simulink model "Main_ekart"  (R2021b)
settings: Solver=FixedStepAuto  StartTime=0.0  StopTime=inf  FixedStep=1/500  RelTol=1e-3  EnableMultiTasking=on
values from neighbouring files (symbols this model uses):
  a = [1 -2.62355180661 2.31468258109 -0.685535977285]    [IMU_filt_100Hz.mat]    (also in IMU_filt_500Hz.mat = [1 -2.92460623545 2.85202781859 -0.92736996835])
  angles = [0 4.9 5 10 15 20 25 30 35 40]    [CreateAllControllers.m]
  b = [0.000699349649901 0.0020980489497 0.0020980489497 0.000699349649901]    [IMU_filt_100Hz.mat]    (also in IMU_filt_500Hz.mat = [6.45184912909e-06 1.93555473873e-05 1.93555473873e-05 6.451)
  D = (DMFx+DMFy)/2    (= 1.2194)    [kart_parameters2.m]
  gear_ratio = 3.2    [kart_parameters2.m]
  L = sys*C    [build_controller_PI.m]    (also in kart_parameters2.m = 1.042)
  newcurrent = [-186.423 -186.283922965 -186.14484593 -186.005768895 -185.866691861 -185.727614826 -185.588537791 -185.449460756 -185.310383721 -185.171306686 -185.032229652 -184.893152617 ... (1000 elements, 1x1000)]    [Torque_map.mat]
  newtorque = [-28.1755 -28.1190925926 -28.0626851852 -28.0062777778 -27.9498703704 -27.893462963 -27.8370555556 -27.7806481481 -27.7242407407 -27.6678333333 -27.6114259259 -27.5550185185 ... (1000 elements, 1x1000)]    [Torque_map.mat]
  percent = [0 0.1001001001 0.2002002002 0.3003003003 0.4004004004 0.500500500501 0.600600600601 0.700700700701 0.800800800801 0.900900900901 1.001001001 1.1011011011 ... (1000 elements, 1x1000)]    [Torque_accel.mat]
  speeds = [0 19.9 20 30 40]    [CreateAllControllers.m]
  table_i = [zeros(1,10) ... (first row only)    [CreateAllControllers.m]
  table_p = [zeros(1, 10) ... (first row only)    [CreateAllControllers.m]
  torque = [0.1025 0.130601101101 0.158702202202 0.186803303303 0.214904404404 0.243005505506 0.271106606607 0.299207707708 0.327308808809 0.35540990991 0.383511011011 0.411612112112 ... (1000 elements, 1x1000)]    [Torque_accel.mat]
libraries: simulink x50, mcp2515lib x46, etargetslib x4, svdutilitieslib x3, cstblocks x2, slpidlib x1
(part 4 of 4)

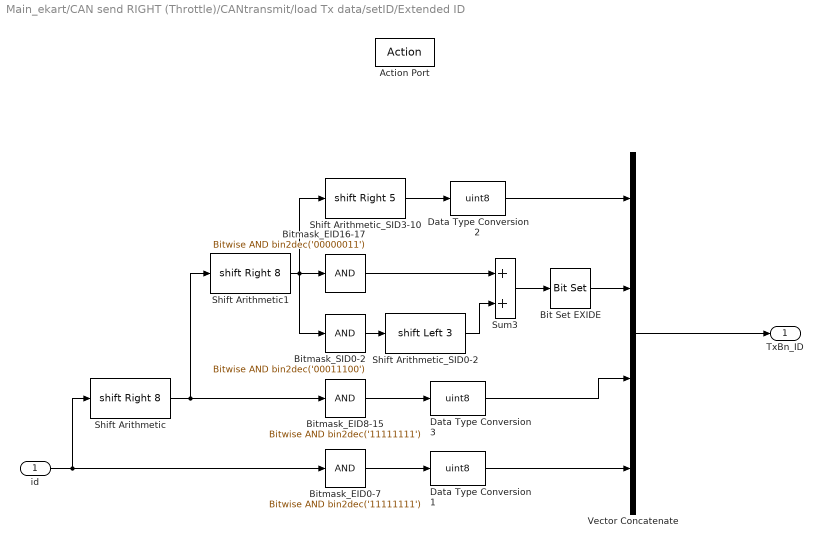
== system Main_ekart/CAN send RIGHT (Throttle)/CANtransmit/load Tx data/setID/Extended ID ==
  id : Inport
  Action Port : ActionPort  ActionPortLabel=if(u1 > 0)
  Bit Set EXIDE : simulink/Logic and Bit Operations/Bit Set  iBit=3
      settings: SourceProductBaseCode=SL
  Bitmask_EID0-7 : simulink/Logic and Bit Operations/Bitwise Operator  logicop=AND  UseBitMask=on  BitMask=bin2dec('11111111')  BitMaskRealWorld=Stored Integer
  Bitmask_EID16-17 : simulink/Logic and Bit Operations/Bitwise Operator  logicop=AND  UseBitMask=on  BitMask=bin2dec('00000011')  BitMaskRealWorld=Stored Integer
  Bitmask_EID8-15 : simulink/Logic and Bit Operations/Bitwise Operator  logicop=AND  UseBitMask=on  BitMask=bin2dec('11111111')  BitMaskRealWorld=Stored Integer
  Bitmask_SID0-2 : simulink/Logic and Bit Operations/Bitwise Operator  logicop=AND  UseBitMask=on  BitMask=bin2dec('00011100')  BitMaskRealWorld=Stored Integer
  Data Type Conversion1 : DataTypeConversion  OutDataTypeStr=uint8  RndMeth=Simplest
  Data Type Conversion2 : DataTypeConversion  OutDataTypeStr=uint8  RndMeth=Simplest
  Data Type Conversion3 : DataTypeConversion  OutDataTypeStr=uint8  RndMeth=Simplest
  Shift Arithmetic : ArithShift  BitShiftNumber=8  BitShiftDirection=Right
  Shift Arithmetic1 : ArithShift  BitShiftNumber=8  BitShiftDirection=Right
  Shift Arithmetic_SID0-2 : ArithShift  BitShiftNumber=3  BitShiftDirection=Left
  Shift Arithmetic_SID3-10 : ArithShift  BitShiftNumber=5  BitShiftDirection=Right
  Sum3 : Sum  OutDataTypeStr=uint8
  Vector Concatenate : Concatenate  NumInputs=4
  TxBn_ID : Outport  VectorParamsAs1DForOutWhenUnconnected=off
  wires:
  Data Type Conversion2/1 -> Vector Concatenate/1
  Shift Arithmetic_SID3-10/1 -> Data Type Conversion2/1
  Bit Set EXIDE/1 -> Vector Concatenate/2
  Shift Arithmetic_SID0-2/1 -> Sum3/2
  Bitmask_SID0-2/1 -> Shift Arithmetic_SID0-2/1
  Bitmask_EID16-17/1 -> Sum3/1
  Sum3/1 -> Bit Set EXIDE/1
  Shift Arithmetic1/1 -> Bitmask_EID16-17/1, Bitmask_SID0-2/1, Shift Arithmetic_SID3-10/1
  Data Type Conversion3/1 -> Vector Concatenate/3
  Bitmask_EID8-15/1 -> Data Type Conversion3/1
  Shift Arithmetic/1 -> Bitmask_EID8-15/1, Shift Arithmetic1/1
  Data Type Conversion1/1 -> Vector Concatenate/4
  Bitmask_EID0-7/1 -> Data Type Conversion1/1
  id/1 -> Bitmask_EID0-7/1, Shift Arithmetic/1
  Vector Concatenate/1 -> TxBn_ID/1

== system Main_ekart/CAN send RIGHT (Throttle)/CANtransmit/load Tx data/setID/Standard ID ==
  id : Inport
  Action Port : ActionPort  ActionPortLabel=else
  Vector Concatenate : Concatenate  NumInputs=4
  convert_ID : Subsystem  TreatAsAtomicUnit=on
  no data : Constant  Value=0  OutDataTypeStr=uint8
  TxBn_ID : Outport  VectorParamsAs1DForOutWhenUnconnected=off
  wires:
  convert_ID/1(SIDH) -> Vector Concatenate/1
  id/1 -> convert_ID/1(id)
  convert_ID/2(SIDL) -> Vector Concatenate/2
  no data/1 -> Vector Concatenate/4, Vector Concatenate/3
  Vector Concatenate/1 -> TxBn_ID/1

== system Main_ekart/Receive_CAN/CANreceive/readRxBuffer/getID/checkExtendedId ==
  SIDL : Inport
  Bitmask_EXIDE : simulink/Logic and Bit Operations/Bitwise Operator  logicop=AND  UseBitMask=on  BitMask=bin2dec('00001000')  BitMaskRealWorld=Stored Integer
  MCP_TXB_EXIDE_M : Constant  Value=hex2dec('08')  OutDataTypeStr=uint8
  Relational Operator : RelationalOperator  Operator===  OutDataTypeStr=boolean  RndMeth=Nearest
  ext : Outport
  wires:
  Relational Operator/1 -> ext/1
  MCP_TXB_EXIDE_M/1 -> Relational Operator/1
  Bitmask_EXIDE/1 -> Relational Operator/2
  SIDL/1 -> Bitmask_EXIDE/1

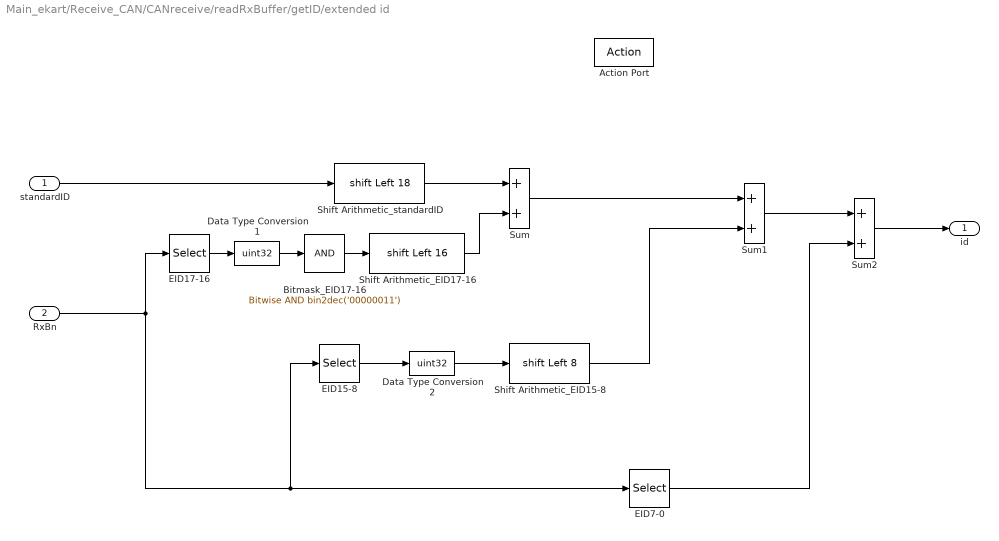
== system Main_ekart/Receive_CAN/CANreceive/readRxBuffer/getID/extended id ==
  standardID : Inport
  RxBn : Inport  Port=2
  Action Port : ActionPort  ActionPortLabel=if(u1 == 1)
  Bitmask_EID17-16 : simulink/Logic and Bit Operations/Bitwise Operator  logicop=AND  UseBitMask=on  BitMask=bin2dec('00000011')  BitMaskRealWorld=Stored Integer
  Data Type Conversion1 : DataTypeConversion  OutDataTypeStr=uint32
  Data Type Conversion2 : DataTypeConversion  OutDataTypeStr=uint32
  EID15-8 : Selector  IndexMode=Zero-based  InputPortWidth=13  IndexOptions=Index vector (dialog)  Indices=2  OutputSizes=1
  EID17-16 : Selector  IndexMode=Zero-based  InputPortWidth=13  IndexOptions=Index vector (dialog)  Indices=1  OutputSizes=1
  EID7-0 : Selector  IndexMode=Zero-based  InputPortWidth=13  IndexOptions=Index vector (dialog)  Indices=3  OutputSizes=1
  Shift Arithmetic_EID15-8 : ArithShift  BitShiftNumber=8  BitShiftDirection=Left
  Shift Arithmetic_EID17-16 : ArithShift  BitShiftNumber=16  BitShiftDirection=Left
  Shift Arithmetic_standardID : ArithShift  BitShiftNumber=18  BitShiftDirection=Left
  Sum : Sum
  Sum1 : Sum
  Sum2 : Sum
  id : Outport
  wires:
  Sum2/1 -> id/1
  standardID/1 -> Shift Arithmetic_standardID/1
  Shift Arithmetic_standardID/1 -> Sum/1
  Shift Arithmetic_EID17-16/1 -> Sum/2
  Sum/1 -> Sum1/1
  Shift Arithmetic_EID15-8/1 -> Sum1/2
  EID15-8/1 -> Data Type Conversion2/1
  Sum1/1 -> Sum2/1
  RxBn/1 -> EID15-8/1, EID7-0/1, EID17-16/1
  EID7-0/1 -> Sum2/2
  EID17-16/1 -> Data Type Conversion1/1
  Data Type Conversion1/1 -> Bitmask_EID17-16/1
  Bitmask_EID17-16/1 -> Shift Arithmetic_EID17-16/1
  Data Type Conversion2/1 -> Shift Arithmetic_EID15-8/1

== system Main_ekart/Receive_CAN/CANreceive/readRxBuffer/getID/getStandardID ==
  SIDL : Inport
  SIDH : Inport  Port=2
  Bitmask_SID2-0 : simulink/Logic and Bit Operations/Bitwise Operator  logicop=AND  UseBitMask=on  BitMask=bin2dec('11100000')  BitMaskRealWorld=Stored Integer
  Data Type Conversion : DataTypeConversion  OutDataTypeStr=uint32
  Shift Arithmetic_SID10-3 : ArithShift  BitShiftNumber=3  BitShiftDirection=Left
  Shift Arithmetic_SID2-0 : ArithShift  BitShiftNumber=5  BitShiftDirection=Right
  Sum1 : Sum
  stadardID : Outport
  wires:
  Sum1/1 -> stadardID/1
  Shift Arithmetic_SID2-0/1 -> Sum1/1
  Shift Arithmetic_SID10-3/1 -> Sum1/2
  SIDL/1 -> Bitmask_SID2-0/1
  SIDH/1 -> Data Type Conversion/1
  Bitmask_SID2-0/1 -> Shift Arithmetic_SID2-0/1
  Data Type Conversion/1 -> Shift Arithmetic_SID10-3/1

== system Main_ekart/Receive_CAN/CANreceive/readRxBuffer/getID/standard id ==
  stadardID : Inport
  Action Port : ActionPort  ActionPortLabel=else
  id : Outport
  wires:
  stadardID/1 -> id/1

== system Main_ekart/CAN send LEFT (Throttle)/CANtransmit/load Tx data/setID/Standard ID/convert_ID ==
  id : Inport
  Bitmask_SID0-10 : simulink/Logic and Bit Operations/Bitwise Operator  logicop=AND  UseBitMask=on  BitMask=bin2dec('0000011111111111')  BitMaskRealWorld=Stored Integer
  Bitmask_SID0-2 : simulink/Logic and Bit Operations/Bitwise Operator  logicop=AND  UseBitMask=on  BitMask=bin2dec('0000000011100000')  BitMaskRealWorld=Stored Integer
  Data Type Conversion1 : DataTypeConversion  OutDataTypeStr=uint8  RndMeth=Simplest
  Data Type Conversion2 : DataTypeConversion  OutDataTypeStr=uint8  RndMeth=Simplest
  Shift Arithmetic1 : ArithShift  BitShiftNumber=3  BitShiftDirection=Right
  Shift Arithmetic2 : ArithShift  BitShiftNumber=5  BitShiftDirection=Left
  SIDH : Outport  VectorParamsAs1DForOutWhenUnconnected=off
  SIDL : Outport  Port=2  VectorParamsAs1DForOutWhenUnconnected=off
  wires:
  Shift Arithmetic1/1 -> Data Type Conversion1/1
  Data Type Conversion1/1 -> SIDH/1
  Bitmask_SID0-10/1 -> Shift Arithmetic2/1, Shift Arithmetic1/1
  Data Type Conversion2/1 -> SIDL/1
  Shift Arithmetic2/1 -> Bitmask_SID0-2/1
  id/1 -> Bitmask_SID0-10/1
  Bitmask_SID0-2/1 -> Data Type Conversion2/1

== system Main_ekart/CAN send LEFT (brake)/CANtransmit/load Tx data/setID/Standard ID/convert_ID ==
  id : Inport
  Bitmask_SID0-10 : simulink/Logic and Bit Operations/Bitwise Operator  logicop=AND  UseBitMask=on  BitMask=bin2dec('0000011111111111')  BitMaskRealWorld=Stored Integer
  Bitmask_SID0-2 : simulink/Logic and Bit Operations/Bitwise Operator  logicop=AND  UseBitMask=on  BitMask=bin2dec('0000000011100000')  BitMaskRealWorld=Stored Integer
  Data Type Conversion1 : DataTypeConversion  OutDataTypeStr=uint8  RndMeth=Simplest
  Data Type Conversion2 : DataTypeConversion  OutDataTypeStr=uint8  RndMeth=Simplest
  Shift Arithmetic1 : ArithShift  BitShiftNumber=3  BitShiftDirection=Right
  Shift Arithmetic2 : ArithShift  BitShiftNumber=5  BitShiftDirection=Left
  SIDH : Outport  VectorParamsAs1DForOutWhenUnconnected=off
  SIDL : Outport  Port=2  VectorParamsAs1DForOutWhenUnconnected=off
  wires:
  Bitmask_SID0-2/1 -> Data Type Conversion2/1
  id/1 -> Bitmask_SID0-10/1
  Shift Arithmetic2/1 -> Bitmask_SID0-2/1
  Data Type Conversion2/1 -> SIDL/1
  Bitmask_SID0-10/1 -> Shift Arithmetic1/1, Shift Arithmetic2/1
  Data Type Conversion1/1 -> SIDH/1
  Shift Arithmetic1/1 -> Data Type Conversion1/1

== system Main_ekart/CAN send RIGHT (Brake)/CANtransmit/load Tx data/setID/Standard ID/convert_ID ==
  id : Inport
  Bitmask_SID0-10 : simulink/Logic and Bit Operations/Bitwise Operator  logicop=AND  UseBitMask=on  BitMask=bin2dec('0000011111111111')  BitMaskRealWorld=Stored Integer
  Bitmask_SID0-2 : simulink/Logic and Bit Operations/Bitwise Operator  logicop=AND  UseBitMask=on  BitMask=bin2dec('0000000011100000')  BitMaskRealWorld=Stored Integer
  Data Type Conversion1 : DataTypeConversion  OutDataTypeStr=uint8  RndMeth=Simplest
  Data Type Conversion2 : DataTypeConversion  OutDataTypeStr=uint8  RndMeth=Simplest
  Shift Arithmetic1 : ArithShift  BitShiftNumber=3  BitShiftDirection=Right
  Shift Arithmetic2 : ArithShift  BitShiftNumber=5  BitShiftDirection=Left
  SIDH : Outport  VectorParamsAs1DForOutWhenUnconnected=off
  SIDL : Outport  Port=2  VectorParamsAs1DForOutWhenUnconnected=off
  wires:
  Shift Arithmetic1/1 -> Data Type Conversion1/1
  Data Type Conversion1/1 -> SIDH/1
  Bitmask_SID0-10/1 -> Shift Arithmetic2/1, Shift Arithmetic1/1
  Data Type Conversion2/1 -> SIDL/1
  Shift Arithmetic2/1 -> Bitmask_SID0-2/1
  id/1 -> Bitmask_SID0-10/1
  Bitmask_SID0-2/1 -> Data Type Conversion2/1

== system Main_ekart/CAN send RIGHT (Throttle)/CANtransmit/load Tx data/setID/Standard ID/convert_ID ==
  id : Inport
  Bitmask_SID0-10 : simulink/Logic and Bit Operations/Bitwise Operator  logicop=AND  UseBitMask=on  BitMask=bin2dec('0000011111111111')  BitMaskRealWorld=Stored Integer
  Bitmask_SID0-2 : simulink/Logic and Bit Operations/Bitwise Operator  logicop=AND  UseBitMask=on  BitMask=bin2dec('0000000011100000')  BitMaskRealWorld=Stored Integer
  Data Type Conversion1 : DataTypeConversion  OutDataTypeStr=uint8  RndMeth=Simplest
  Data Type Conversion2 : DataTypeConversion  OutDataTypeStr=uint8  RndMeth=Simplest
  Shift Arithmetic1 : ArithShift  BitShiftNumber=3  BitShiftDirection=Right
  Shift Arithmetic2 : ArithShift  BitShiftNumber=5  BitShiftDirection=Left
  SIDH : Outport  VectorParamsAs1DForOutWhenUnconnected=off
  SIDL : Outport  Port=2  VectorParamsAs1DForOutWhenUnconnected=off
  wires:
  Bitmask_SID0-2/1 -> Data Type Conversion2/1
  id/1 -> Bitmask_SID0-10/1
  Shift Arithmetic2/1 -> Bitmask_SID0-2/1
  Data Type Conversion2/1 -> SIDL/1
  Bitmask_SID0-10/1 -> Shift Arithmetic1/1, Shift Arithmetic2/1
  Data Type Conversion1/1 -> SIDH/1
  Shift Arithmetic1/1 -> Data Type Conversion1/1

== matlab function Main_ekart/Torque Allocation (Low-Level Controller)/MATLAB Function ==
  data: TRL output; deltaT input; Tdem input; TRR output
function [TRL, TRR] = fcn(deltaT, Tdem)

   
    TRL = Tdem/2 - deltaT;
    TRR = Tdem/2 + deltaT;


end

== matlab function Main_ekart/Convert to Brake or Throttle Current1/MATLAB Function1 ==
  data: sign_current input; brake_current output; current input; throttle_current output
function [brake_current, throttle_current] = fcn(sign_current, current)

    if(sign_current==1)
        brake_current = abs(current);
        throttle_current = 0;
    else
        brake_current = 0;
        throttle_current = current;
    end

== matlab function Main_ekart/Receive_CAN/Subsystem7/MATLAB Function ==
  data: A input; B output
function B = flip_array(A)

B = flip(A);

end

== matlab function Main_ekart/Ref Gen/reference gen ==
  data: u input; deltaSW input; r_ref output; L input; D input
function r_ref = fcn(u, deltaSW, L, D)

steer_ratio = 2;

delta = 1/steer_ratio*deltaSW;

% r_ref = 1.2*u*delta/(lf+lr);
g = 9.81;
K = -0.00;
r_ref = u*delta/(L + u^2*K);

r_max = D*g/u;

r_ref = sign(r_ref)*min(abs(r_ref),r_max);

== matlab function Main_ekart/Receive_CAN/Subsystem1/MATLAB Function ==
  data: A input; B output
function B = flip_array(A)

B = flip(A);

end

== matlab function Main_ekart/Receive_CAN/Subsystem5/MATLAB Function ==
  data: A input; B output
function B = flip_array(A)

B = flip(A);

end

== matlab function Main_ekart/Receive_CAN/Subsystem3/MATLAB Function ==
  data: Valpi_2 input; steering_angle_rad output; steering_pot_raw input; Valnegpi_2 input
function steering_angle_rad = fcn(Valpi_2, steering_pot_raw, Valnegpi_2)
    
    
    m = pi/(Valpi_2-Valnegpi_2);
    p = pi/2-m*Valpi_2;
    
    steering_angle_rad = m*steering_pot_raw+p;

    if(steering_angle_rad<-pi/2)
        steering_angle_rad = -single(pi/2);
    else 
        if(steering_angle_rad>pi/2)
            steering_angle_rad = single(pi/2);
        end
    end
end

== matlab function Main_ekart/Receive_CAN/Subsystem4/MATLAB Function ==
  data: Val100 input; throttle_percent output; throttle_pot_raw input; Val0 input
function throttle_percent = fcn(Val100, throttle_pot_raw, Val0)
    
    
    m = 100/(Val100-Val0);
    p = 100-m*Val100;
    
   throttle_percent = m*single(throttle_pot_raw)+p;

    if(throttle_percent<0)
        throttle_percent = single(0);
    else 
        if(throttle_percent>100)
            throttle_percent = single(100);
        end
    end
end

== matlab function Main_ekart/CAN send LEFT (brake)/MATLAB Function ==
  data: A input; B output
function B = flip_array(A)

B = flip(A);

end

== matlab function Main_ekart/CAN send RIGHT (Brake)/MATLAB Function ==
  data: A input; B output
function B = flip_array(A)

B = flip(A);

end

== matlab function Main_ekart/CAN send LEFT (Throttle)/MATLAB Function ==
  data: A input; B output
function B = flip_array(A)

B = flip(A);

end

== matlab function Main_ekart/Convert to Brake or Throttle Current/MATLAB Function1 ==
  data: sign_current input; brake_current output; current input; throttle_current output
function [brake_current, throttle_current] = fcn(sign_current, current)

    if(sign_current==1)
        brake_current = abs(current);
        throttle_current = 0;
    else
        brake_current = 0;
        throttle_current = current;
    end

== matlab function Main_ekart/CAN send RIGHT (Throttle)/MATLAB Function ==
  data: A input; B output
function B = flip_array(A)

B = flip(A);

end
